simulink model "klassisk_lin"  (Simulink 2.20)
settings: Solver=ode45  StartTime=0.0  StopTime=10  RelTol=1e-3  AbsTol=1e-6
libraries: simulink_extras x3, simulink x1
settings Model: ConsistencyChecking=off  RTWPlaceOutputsASAP=off

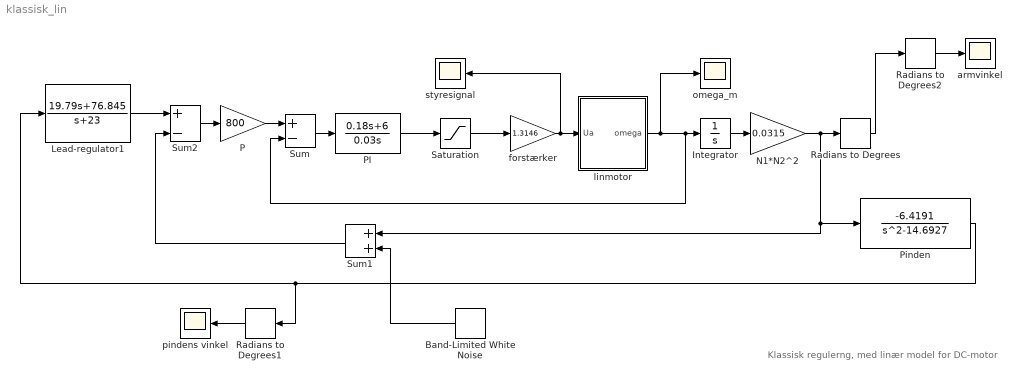
== system klassisk_lin ==
  note: Klassisk regulerng, med linær model for DC-motor
  Band-Limited White Noise : simulink/Sources/Band-Limited White Noise  Orientation=left  Cov=[0.0000001]  Ts=0.001  seed=[23341]
  Integrator : Integrator  ExternalReset=none  InitialConditionSource=internal  InitialCondition=0  LimitOutput=off  UpperSaturationLimit=inf  LowerSaturationLimit=-inf  ShowSaturationPort=off  ShowStatePort=off  AbsoluteTolerance=auto
  Lead-regulator1 : TransferFcn  Numerator=[19.79 76.845]  Denominator=[1 23]
  N1*N2^2 : Gain  Gain=0.0315
  P : Gain  Gain=800
  PI : TransferFcn  Numerator=[0.18 6]  Denominator=[0.03 0]
  Pinden : TransferFcn  Numerator=[-6.4191]  Denominator=[1 0 -14.6927 ]
  Radians to Degrees : simulink_extras/Transformations/Radians to Degrees
  Radians to Degrees1 : simulink_extras/Transformations/Radians to Degrees  Orientation=left
  Radians to Degrees2 : simulink_extras/Transformations/Radians to Degrees
  Saturation : Saturate  UpperLimit=5  LowerLimit=-5
  Sum : Sum  Inputs=+-
  Sum1 : Sum  Orientation=left  Inputs=++
  Sum2 : Sum  Inputs=+-
  armvinkel : Scope
      settings: TickLabels=on  TimeRange=10  YMin=-0.225  YMax=0.275  SaveToWorkspace=off  SaveName=ScopeData  LimitMaxRows=off
  forstærker : Gain  Gain=1.3146
  linmotor : Subsystem
  "omega_m " : Scope
      settings: TickLabels=on  TimeRange=10  YMin=-0.00065  YMax=0  SaveToWorkspace=off  SaveName=ScopeData
  pindens vinkel : Scope
      settings: TickLabels=on  TimeRange=5  YMin=-0.045  YMax=0.03  SaveToWorkspace=off  SaveName=ScopeData  LimitMaxRows=off
  styresignal : Scope
      settings: TickLabels=on  TimeRange=0.5  YMin=0  YMax=13  SaveToWorkspace=off  SaveName=ScopeData
  wires:
  Sum/1 -> PI/1
  Saturation/1 -> forstærker/1
  forstærker/1 -> styresignal/1, linmotor/1(Ua)
  Integrator/1 -> N1*N2^2/1
  PI/1 -> Saturation/1
  N1*N2^2/1 -> Radians to Degrees/1, Pinden/1, Sum1/1
  linmotor/1(omega) -> "omega_m "/1, Integrator/1, Sum/2
  P/1 -> Sum/1
  Sum2/1 -> P/1
  Pinden/1 -> Radians to Degrees1/1, Lead-regulator1/1
  Band-Limited White Noise/1 -> Sum1/2
  Radians to Degrees/1 -> Radians to Degrees2/1
  Radians to Degrees2/1 -> armvinkel/1
  Sum1/1 -> Sum2/2
  Lead-regulator1/1 -> Sum2/1
  Radians to Degrees1/1 -> pindens vinkel/1

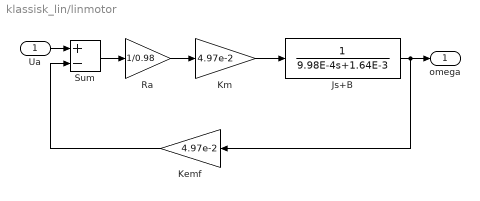
== system klassisk_lin/linmotor ==
  Ua : Inport  Port=1  PortWidth=-1  SampleTime=-1
  Js+B : TransferFcn  Numerator=[1]  Denominator=[9.98E-4 1.64E-3]
  Kemf : Gain  Orientation=left  Gain=4.97e-2
  Km : Gain  Gain=4.97e-2
  Ra : Gain  Gain=1/0.98
  Sum : Sum  Inputs=+-
  omega : Outport  Port=1  InitialOutput=0
  wires:
  Ra/1 -> Km/1
  Sum/1 -> Ra/1
  Kemf/1 -> Sum/2
  Js+B/1 -> Kemf/1, omega/1
  Ua/1 -> Sum/1
  Km/1 -> Js+B/1
